simulink model "dnrdt"  (R2021a)
settings: Solver=VariableStepAuto  StartTime=0.0  StopTime=200  RelTol=1e-3
values from neighbouring files (symbols this model uses):
  alpha_c = 0.00001    (= 1e-05)    [full_plant.m]    (also in full_plant_20.m; policy.m; reactor_core.m)
  alpha_f = -0.00005    (= -5e-05)    [full_plant.m]    (also in full_plant_20.m; policy.m; reactor_core.m)
  beta = p ^ 0.25    (= 0)    [XSteam.m]    (also in XSteam_h_ps.m; full_plant.m = sum(betas); full_plant_20.m = sum(betas); policy.m = sum(betas))
  betas = [0.000215; 0.001424; 0.001274; 0.002568; 0.000748; 0.000273]    [full_plant.m]    (also in full_plant_20.m; policy.m; reactor_core.m)
  ff = 0.98    [full_plant.m]    (also in full_plant_20.m; policy.m; reactor_core.m)
  Gr = 0.0001 * beta    [full_plant_20.m]    (also in reactor_core.m = 0.00001 * beta)
  Lambda = 0.0001    [full_plant.m]    (also in full_plant_20.m; policy.m; reactor_core.m)
  lambdas = [0.0124; 0.0305; 0.1110; 0.3010; 1.1400; 3.0100]    [full_plant.m]    (also in full_plant_20.m; policy.m; reactor_core.m)
  M = M_sg * 2    (= 92.7075812274)    [full_plant.m]    (also in full_plant_20.m; policy.m; reactor_core.m)
  mu_c = 70.5    [full_plant.m]    (also in full_plant_20.m; policy.m; reactor_core.m)
  mu_f = 26.3    [full_plant.m]    (also in full_plant_20.m; policy.m; reactor_core.m)
  Omega = P_thermal0 * ff / (T_f0 - T_h0)    (= 6.72125630959)    [full_plant.m]    (also in full_plant_20.m; policy.m; reactor_core.m)
  P_thermal0 = 2568    [full_plant.m]    (also in full_plant_20.m; policy.m; reactor_core.m; sg.m)
  T_c0 = 290.0    (= 290)    [full_plant.m]    (also in full_plant_20.m; policy.m; reactor_core.m; sg.m)
  T_f0 = 965.28 - 273.15    (= 692.13)    [full_plant.m]    (also in full_plant_20.m; policy.m; reactor_core.m)
  T_h0 = 317.7    [full_plant.m]    (also in full_plant_20.m; policy.m; reactor_core.m; sg.m)
  T_sg_out0 = XSteam('Tsat_p', P_sg0 * 10)    [full_plant.m]    (also in full_plant_20.m; policy.m; reactor_core.m; sg.m)
  Z1 = P_thermal0 / (T_p0 - T_m0) / num_sg    [full_plant.m]    (also in full_plant_20.m = P_thermal0 / (T_c0 - T_m0) / num_sg; policy.m; reactor_core.m; sg.m)
  Z2 = P_thermal0 / (T_m0 - T_sg_out0) / num_sg    [full_plant.m]    (also in full_plant_20.m; policy.m; reactor_core.m; sg.m)
libraries: simulink x1
settings Model: Creator=xxc90  LastModifiedBy=xxc90

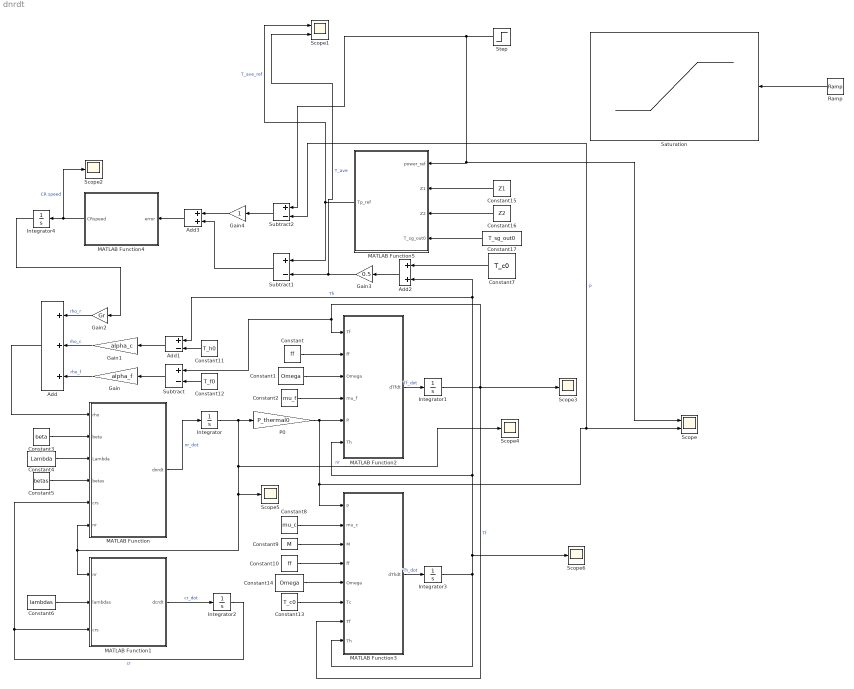
== system dnrdt ==
  Add : Sum  Inputs=+++
  Add1 : Sum  Inputs=+-
  Add2 : Sum
  Add3 : Sum
  Constant : Constant  Value=ff
  Constant1 : Constant  Value=Omega
  Constant10 : Constant  Value=ff
  Constant11 : Constant  Value=T_h0
  Constant12 : Constant  Value=T_f0
  Constant13 : Constant  Value=T_c0
  Constant14 : Constant  Value=Omega
  Constant15 : Constant  Value=Z1
  Constant16 : Constant  Value=Z2
  Constant17 : Constant  Value=T_sg_out0
  Constant2 : Constant  Value=mu_f
  Constant3 : Constant  Value=beta
  Constant4 : Constant  Value=Lambda
  Constant5 : Constant  Value=betas
  Constant6 : Constant  Value=lambdas
  Constant7 : Constant  Value=T_c0
  Constant8 : Constant  Value=mu_c
  Constant9 : Constant  Value=M
  Gain : Gain  Gain=alpha_f
  Gain1 : Gain  Gain=alpha_c
  Gain2 : Gain  Gain=Gr
  Gain3 : Gain  Gain=0.5
  Gain4 : Gain
  Integrator : Integrator  InitialCondition=1
  Integrator1 : Integrator  InitialCondition=T_f0
  Integrator2 : Integrator  InitialCondition=[1;1;1;1;1;1]
  Integrator3 : Integrator  InitialCondition=T_h0
  Integrator4 : Integrator
  MATLAB Function : MATLAB Function  TreatAsAtomicUnit=on
  MATLAB Function1 : MATLAB Function  TreatAsAtomicUnit=on
  MATLAB Function2 : MATLAB Function  TreatAsAtomicUnit=on
  MATLAB Function3 : MATLAB Function  TreatAsAtomicUnit=on
  MATLAB Function4 : MATLAB Function  TreatAsAtomicUnit=on
  MATLAB Function5 : MATLAB Function  TreatAsAtomicUnit=on
  P0 : Gain  Gain=P_thermal0
  Ramp : simulink/Sources/Ramp  slope=2.14  start=10  InitialOutput=P_thermal0
  Saturation : Saturate  UpperLimit=P_thermal0 * 1.1
  Scope : Scope  NumInputPorts=2
  Scope1 : Scope  NumInputPorts=2
  Scope{2..6} (5 alike) : Scope
  Step : Step  Before=P_thermal0  After=P_thermal0 *1.1  SampleTime=0
  Subtract : Sum  Inputs=+-
  Subtract1 : Sum  Inputs=+-
  Subtract2 : Sum  Inputs=+-
  wires:
  MATLAB Function/1(dnrdt) -> Integrator/1  "nr_dot"
  Integrator/1 -> P0/1, Scope4/1, Scope5/1, MATLAB Function/6(nr), MATLAB Function1/1(nr)  "nr"
  P0/1 -> Subtract2/2, Scope/2, MATLAB Function3/1(P), MATLAB Function2/5(P)  "P"
  MATLAB Function2/1(dTfdt) -> Integrator1/1  "Tf_dot"
  Integrator1/1 -> Scope3/1, MATLAB Function3/7(Tf), Subtract/1, MATLAB Function2/1(Tf)  "Tf"
  Constant/1 -> MATLAB Function2/2(ff)
  Constant1/1 -> MATLAB Function2/3(Omega)
  Constant2/1 -> MATLAB Function2/4(mu_f)
  Constant3/1 -> MATLAB Function/2(beta)
  Constant4/1 -> MATLAB Function/3(Lambda)
  Constant5/1 -> MATLAB Function/4(betas)
  MATLAB Function1/1(dcrdt) -> Integrator2/1  "cr_dot"
  Integrator2/1 -> MATLAB Function/5(crs), MATLAB Function1/3(crs)  "cr"
  Constant6/1 -> MATLAB Function1/2(lambdas)
  MATLAB Function3/1(dThdt) -> Integrator3/1  "Th_dot"
  Integrator3/1 -> Scope6/1, MATLAB Function2/6(Th), Add2/2, Add1/1, MATLAB Function3/8(Th)  "Th"
  Constant8/1 -> MATLAB Function3/2(mu_c)
  Constant9/1 -> MATLAB Function3/3(M)
  Constant10/1 -> MATLAB Function3/4(ff)
  Add/1 -> MATLAB Function/1(rho)
  Subtract/1 -> Gain/1
  Gain/1 -> Add/3  "rho_f"
  Add1/1 -> Gain1/1
  Gain1/1 -> Add/2  "rho_c"
  Constant13/1 -> MATLAB Function3/6(Tc)
  Constant14/1 -> MATLAB Function3/5(Omega)
  Gain2/1 -> Add/1  "rho_r"
  Constant7/1 -> Add2/1
  Add2/1 -> Gain3/1
  Gain3/1 -> Scope1/2, Subtract1/2  "T_ave"
  MATLAB Function5/1(Tp_ref) -> Subtract1/1, Scope1/1  "T_ave_ref"
  Subtract1/1 -> Add3/2
  Constant15/1 -> MATLAB Function5/2(Z1)
  Constant16/1 -> MATLAB Function5/3(Z2)
  Constant17/1 -> MATLAB Function5/4(T_sg_out0)
  Ramp/1 -> Saturation/1
  Integrator4/1 -> Gain2/1
  MATLAB Function4/1(CRspeed) -> Scope2/1, Integrator4/1  "CR speed"
  Add3/1 -> MATLAB Function4/1(error)
  Constant12/1 -> Subtract/2
  Constant11/1 -> Add1/2
  Gain4/1 -> Add3/1
  Subtract2/1 -> Gain4/1
  Step/1 -> Scope/1, MATLAB Function5/1(power_ref), Subtract2/1

== matlab function dnrdt/MATLAB Function1 ==
  data: nr input; lambdas input; dcrdt output; crs input
function dcrdt = dcrdt(nr, lambdas, crs)
    dcrdt = lambdas * nr - lambdas .* crs;
end

== matlab function dnrdt/MATLAB Function ==
  data: rho input; dnrdt output size=1; beta input; Lambda input; betas input; crs input; nr input
function dnrdt= dnrdt(rho, beta, Lambda, betas, crs, nr)
    dnrdt = (rho - beta) / Lambda * nr + betas' / Lambda * crs;
end

== matlab function dnrdt/MATLAB Function2 ==
  data: Tf input; ff input; Omega input; mu_f input; P input; Th input; dTfdt output
function dTfdt = dTfdt(Tf, ff, Omega, mu_f, P, Th)
    dTfdt = (ff * P - Omega *(Tf - Th)) / mu_f
end

== matlab function dnrdt/MATLAB Function3 ==
  data: P input; dThdt output; mu_c input; M input; ff input; Omega input; Tc input; Tf input; Th input
function dThdt = dThdt(P, mu_c, M, ff, Omega, Tc, Tf, Th)
    dThdt = ((1-ff)*P + Omega*(Tf-Th) - M*(Th - Tc)) / mu_c
end

== matlab function dnrdt/MATLAB Function4 ==
  data: error input; CRspeed output
function CRspeed = CRspeed(error)
    error_F = error * 9 / 5;
    if error_F < -5
        CRspeed = -72;
    elseif (error_F >= -5) && (error_F<=-3)
        CRspeed = 88 + 32 * error_F;
    elseif (error_F > -3) && (error_F<-1)
        CRspeed = -8;
    elseif (error_F >= -1) && (error_F<= 1)
        CRspeed = 0;
    elseif (error_F > 1) && (error_F<3)
        CRspeed = 8;
    elseif (error_F >= 3) && (error_F<=5)
        CRspeed = -88 + 32 * error_F;
    else
        CRspeed = 72
end

== matlab function dnrdt/MATLAB Function5 ==
  data: power_ref input; Tp_ref output; Z1 input; Z2 input; T_sg_out0 input
function Tp_ref = Tp_ref(power_ref, Z1, Z2, T_sg_out0)
    Tp_ref = power_ref / Z1 / 2 + power_ref / Z2 / 2 + T_sg_out0;
end
